simulink model "switch_inductor_system"  (R2025b)
settings: Solver=ode23t  StartTime=0.0  StopTime=10e-6  MaxStep=1e-8  RelTol=1e-4
libraries: fl_lib x93, nesl_utility x82, eeGeneralControl x28, batteryecm_lib x17, eePwmGenerator x11, slpidlib x9, simulink x2, slctrl_fre x1
(part 3 of 3)

== system switch_inductor_system/Feedback_BC6 ==
  u : Inport
  Constant7 : Constant  Value=0.5
  PID Controller1 : slpidlib/PID Controller  Controller=PI  Form=Parallel  TimeDomain=Discrete-time  UseExternalTs=off  SampleTime=1e-5  IntegratorMethod=Forward Euler  FilterMethod=Forward Euler  ControllerParametersSource=internal  P=1  I=3  UseKiTs=off  D=0  UseExternalDerivativeSource=off  N=100  UseFilter=on  TunerSelectOption=Transfer Function Based (PID Tuner App)  InitialConditionSource=internal  InitialConditionForIntegrator=0  InitialConditionForFilter=0  DifferentiatorICPrevScaledInput=0  ExternalReset=none  TrackingMode=off  Kt=1  LimitOutput=on  SatLimitsSource=internal  UpperSaturationLimit=0.5  LowerSaturationLimit=-0.5  LinearizeAsGain=on  AntiWindupMode=clamping  Kb=1  LimitIntegrator=off  UpperIntegratorSaturationLimit=inf  LowerIntegratorSaturationLimit=-inf  POutMin=[]  POutMax=[]  IOutMin=[]  IOutMax=[]  DOutMin=[]  DOutMax=[]  NOutMin=[]  NOutMax=[]  SumOutMin=[]  SumOutMax=[]  SaturationOutMin=[]  SaturationOutMax=[]  PParamMin=[]  PParamMax=[]  IParamMin=[]  IParamMax=[]  DParamMin=[]  DParamMax=[]  NParamMin=[]  NParamMax=[]  KbParamMin=[]  KbParamMax=[]  KtParamMin=[]  KtParamMax=[]  KbOutMin=[]  KbOutMax=[]  KtOutMin=[]  KtOutMax=[]  IntegratorOutMin=[]  IntegratorOutMax=[]  FilterOutMin=[]  FilterOutMax=[]  SumI1OutMin=[]  SumI1OutMax=[]  SumI2OutMin=[]  SumI2OutMax=[]  SumI3OutMin=[]  SumI3OutMax=[]  SumI4OutMin=[]  SumI4OutMax=[]  SumDOutMin=[]  SumDOutMax=[]  DifferentiatorOutMin=[]  DifferentiatorOutMax=[]  FilterDiffOutCoefMin=[]  FilterDiffOutCoefMax=[]  ReciprocalOutMin=[]  ReciprocalOutMax=[]  SumDenOutMin=[]  SumDenOutMax=[]  SumNumOutMin=[]  SumNumOutMax=[]  DivideOutMin=[]  DivideOutMax=[]  UdiffTsProdOutMin=[]  UdiffTsProdOutMax=[]  NTsProdOutMin=[]  NTsProdOutMax=[]  UintegralTsProdOutMin=[]  UintegralTsProdOutMax=[]  UngainTsProdOutMin=[]  UngainTsProdOutMax=[]  ClampingZeroOutDataTypeStr=Inherit: Inherit via back propagation  ClampingZeroOutMin=[]  ClampingZeroOutMax=[]  FilterDenConstantOutDataTypeStr=Inherit: Inherit via back propagation  FilterDenConstantOutMin=[]  FilterDenConstantOutMax=[]  PCopyOutDataTypeStr=Inherit: Inherit via back propagation  PCopyOutMin=[]  PCopyOutMax=[]  NCopyOutDataTypeStr=Inherit: Inherit via back propagation  NCopyOutMin=[]  NCopyOutMax=[]  IntegratorContinuousStateAttributes=''  IntegratorStateMustResolveToSignalObject=off  IntegratorRTWStateStorageClass=Auto  FilterContinuousStateAttributes=''  FilterStateMustResolveToSignalObject=off  FilterRTWStateStorageClass=Auto  ParallelPVariant=InternalParameters  IdealPVariant=Disabled  IVariant=InternalParameters  DVariant=Disabled  IntegratorVariant=Discrete  SatVariant=Enabled  AWVariant=DiscClampingParallel  PCopyVariant=Disabled  TRVariant=Disabled  FdbkBlocksVariant=Forward  IdealPFdbkVariant=Disabled  SatFdbkVariant=Disabled  DerivativeFilterVariant=Disabled  NVariant=Disabled  NCopyVariant=Disabled_SignalSpec  FilterICVariant=Disabled  IntegratorICVariant=InternalICs  ExternalResetVariant=Disabled  TRSumVariant=Passthrough  SumFdbkVariant=Disabled  SumVariant=Sum_PI  TsampFilterVariant=InternalTs  TsampNgainVariant=Passthrough  TsampIntegralVariant=Disabled_SignalSpec  ExternalSaturationOutDataTypeStr=Inherit: Same as second input  DerivativeSourceVariant=Disabled  PreIntVariant=InternalPreInt
  PWM Generator : eePwmGenerator/PWM Generator  CarrCount=Up  Tper=1e-5  Tdelay=0  Ts=1e-8
  Saturation1 : Saturate  UpperLimit=0.8  LowerLimit=0.2
  Scope10 : Scope
      settings: DataLoggingVariableName=ScopeData10
  Scope9 : Scope
      settings: ActiveDisplayYMinimum=0.37658910329171397  ActiveDisplayYMaximum=0.57295686719636774  DataLoggingVariableName=ScopeData9
  Sum7 : Sum  Inputs=|++
  Unit Delay : UnitDelay  InitialCondition=0.5  SampleTime=1e-5  HasFrameUpgradeWarning=on
  PWM : Outport
  wires:
  PID Controller1/1 -> Scope10/1, Sum7/1
  u/1 -> PID Controller1/1
  Constant7/1 -> Sum7/2
  Unit Delay/1 -> Scope9/1, PWM Generator/1
  Saturation1/1 -> Unit Delay/1
  PWM Generator/1 -> PWM/1
  Sum7/1 -> Saturation1/1

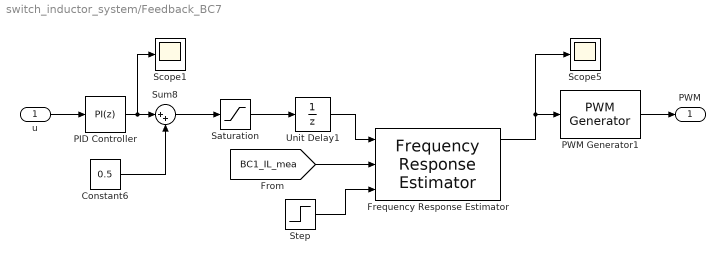
== system switch_inductor_system/Feedback_BC7 ==
  u : Inport
  Constant6 : Constant  Value=0.5
  Frequency Response Estimator : slctrl_fre/Frequency Response Estimator  DiscreteTs=1e-5  OutputMode=control action + perturbation  BlockDataType=double  SineSource=Block parameters  Frequencies=2*pi*logspace(0, 4, 35)  FreqUnits=rad/s  Amplitudes=0.004  NumOfFreq=3  ExperimentMode=Sinestream  NumOfSetPeriod=4  NumOfEstPeriod=6  NumOfSlowestPeriod=3  NumOfPRBSPeriod=1  UseAutogenNumOfPRBSPeriod=off  PRBSSignalOrder=12  UseAutogenPRBSSignalOrder=off  EstimationMode=Online  UseBodePlot=on  BaselinePlant=[]  PlotRefreshFactor=10000  UseExternalTs=off  BodePlotChoice=VariantBode  ExperimentChoice=VariantSS  OutputChoice=VariantCandD  CompiledTsChoice=InternalTs
      settings: LibrarySourceBlock=slctrlblks/Frequency Response Estimation/Frequency Response Estimator
  PID Controller : slpidlib/PID Controller  Controller=PI  Form=Parallel  TimeDomain=Discrete-time  UseExternalTs=off  SampleTime=1e-5  IntegratorMethod=Forward Euler  FilterMethod=Forward Euler  ControllerParametersSource=internal  P=1  I=3  UseKiTs=off  D=0  UseExternalDerivativeSource=off  N=100  UseFilter=on  TunerSelectOption=Transfer Function Based (PID Tuner App)  InitialConditionSource=internal  InitialConditionForIntegrator=0  InitialConditionForFilter=0  DifferentiatorICPrevScaledInput=0  ExternalReset=none  TrackingMode=off  Kt=1  LimitOutput=on  SatLimitsSource=internal  UpperSaturationLimit=0.5  LowerSaturationLimit=-0.5  LinearizeAsGain=on  AntiWindupMode=clamping  Kb=1  LimitIntegrator=off  UpperIntegratorSaturationLimit=inf  LowerIntegratorSaturationLimit=-inf  POutMin=[]  POutMax=[]  IOutMin=[]  IOutMax=[]  DOutMin=[]  DOutMax=[]  NOutMin=[]  NOutMax=[]  SumOutMin=[]  SumOutMax=[]  SaturationOutMin=[]  SaturationOutMax=[]  PParamMin=[]  PParamMax=[]  IParamMin=[]  IParamMax=[]  DParamMin=[]  DParamMax=[]  NParamMin=[]  NParamMax=[]  KbParamMin=[]  KbParamMax=[]  KtParamMin=[]  KtParamMax=[]  KbOutMin=[]  KbOutMax=[]  KtOutMin=[]  KtOutMax=[]  IntegratorOutMin=[]  IntegratorOutMax=[]  FilterOutMin=[]  FilterOutMax=[]  SumI1OutMin=[]  SumI1OutMax=[]  SumI2OutMin=[]  SumI2OutMax=[]  SumI3OutMin=[]  SumI3OutMax=[]  SumI4OutMin=[]  SumI4OutMax=[]  SumDOutMin=[]  SumDOutMax=[]  DifferentiatorOutMin=[]  DifferentiatorOutMax=[]  FilterDiffOutCoefMin=[]  FilterDiffOutCoefMax=[]  ReciprocalOutMin=[]  ReciprocalOutMax=[]  SumDenOutMin=[]  SumDenOutMax=[]  SumNumOutMin=[]  SumNumOutMax=[]  DivideOutMin=[]  DivideOutMax=[]  UdiffTsProdOutMin=[]  UdiffTsProdOutMax=[]  NTsProdOutMin=[]  NTsProdOutMax=[]  UintegralTsProdOutMin=[]  UintegralTsProdOutMax=[]  UngainTsProdOutMin=[]  UngainTsProdOutMax=[]  ClampingZeroOutDataTypeStr=Inherit: Inherit via back propagation  ClampingZeroOutMin=[]  ClampingZeroOutMax=[]  FilterDenConstantOutDataTypeStr=Inherit: Inherit via back propagation  FilterDenConstantOutMin=[]  FilterDenConstantOutMax=[]  PCopyOutDataTypeStr=Inherit: Inherit via back propagation  PCopyOutMin=[]  PCopyOutMax=[]  NCopyOutDataTypeStr=Inherit: Inherit via back propagation  NCopyOutMin=[]  NCopyOutMax=[]  IntegratorContinuousStateAttributes=''  IntegratorStateMustResolveToSignalObject=off  IntegratorRTWStateStorageClass=Auto  FilterContinuousStateAttributes=''  FilterStateMustResolveToSignalObject=off  FilterRTWStateStorageClass=Auto  ParallelPVariant=InternalParameters  IdealPVariant=Disabled  IVariant=InternalParameters  DVariant=Disabled  IntegratorVariant=Discrete  SatVariant=Enabled  AWVariant=DiscClampingParallel  PCopyVariant=Disabled  TRVariant=Disabled  FdbkBlocksVariant=Forward  IdealPFdbkVariant=Disabled  SatFdbkVariant=Disabled  DerivativeFilterVariant=Disabled  NVariant=Disabled  NCopyVariant=Disabled_SignalSpec  FilterICVariant=Disabled  IntegratorICVariant=InternalICs  ExternalResetVariant=Disabled  TRSumVariant=Passthrough  SumFdbkVariant=Disabled  SumVariant=Sum_PI  TsampFilterVariant=InternalTs  TsampNgainVariant=Passthrough  TsampIntegralVariant=Disabled_SignalSpec  ExternalSaturationOutDataTypeStr=Inherit: Same as second input  DerivativeSourceVariant=Disabled  PreIntVariant=InternalPreInt
  PWM Generator1 : eePwmGenerator/PWM Generator  CarrCount=Up  Tper=1e-5  Tdelay=0  Ts=1e-8
  Saturation : Saturate  UpperLimit=0.8  LowerLimit=0.2
  Scope1 : Scope
      settings: ActiveDisplayYMinimum=-0.042552531642600082  ActiveDisplayYMaximum=0.10471177602951695
  Scope5 : Scope
      settings: ActiveDisplayYMinimum=0.39070761591509251  ActiveDisplayYMaximum=0.50905716116304278  DataLoggingVariableName=ScopeData3
  Step : Step  Time=0.5  SampleTime=0
  Sum8 : Sum  Inputs=|++
  Unit Delay1 : UnitDelay  InitialCondition=0.5  SampleTime=1e-5  HasFrameUpgradeWarning=on
  PWM : Outport
  wires:
  Sum8/1 -> Saturation/1
  PID Controller/1 -> Scope1/1, Sum8/1
  Constant6/1 -> Sum8/2
  Saturation/1 -> Unit Delay1/1
  u/1 -> PID Controller/1
  PWM Generator1/1 -> PWM/1
  Unit Delay1/1 -> Frequency Response Estimator/1
  Frequency Response Estimator/1 -> Scope5/1, PWM Generator1/1
  [BC1_IL_mea] -> Frequency Response Estimator/2
  Step/1 -> Frequency Response Estimator/3

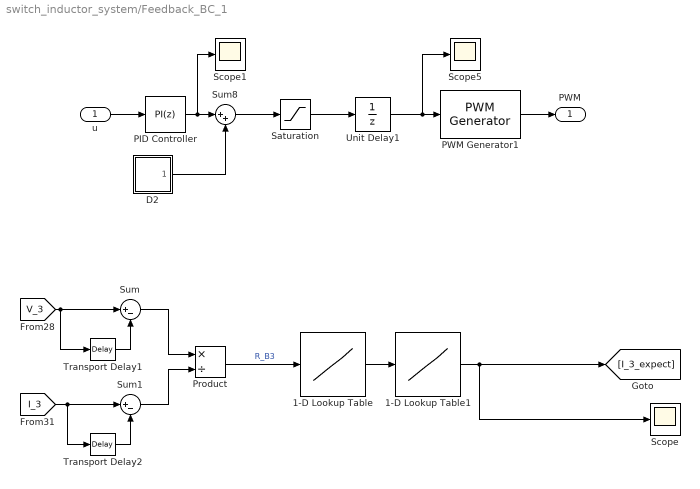
== system switch_inductor_system/Feedback_BC_1 ==
  u : Inport
  1-D Lookup Table : Lookup_n-D  NumberOfTableDimensions=1  BreakpointsForDimension1=[0.005 0.0055 0.006 0.0065 0.007 0.0075 0.008 0.008500000000000001 0.008999999999999999 0.0095 0.01]  Table=[100 90 80 70 60 50 40 30 20 10 5]  InternalRulePriority=Speed  RndMeth=Simplest
  1-D Lookup Table1 : Lookup_n-D  NumberOfTableDimensions=1  BreakpointsForDimension1=[5 10 20 30 40 50 60 70 80 90 100]  Table=[0.6 0.7 0.7125 0.725 0.75 0.8 0.9 1 1.1 1.2 1.3]  InternalRulePriority=Speed  RndMeth=Simplest
  D2 : Subsystem
  PID Controller : slpidlib/PID Controller  Controller=PI  Form=Parallel  TimeDomain=Discrete-time  UseExternalTs=off  SampleTime=1e-5  IntegratorMethod=Forward Euler  FilterMethod=Forward Euler  ControllerParametersSource=internal  P=1  I=3  UseKiTs=off  D=0  UseExternalDerivativeSource=off  N=100  UseFilter=on  TunerSelectOption=Transfer Function Based (PID Tuner App)  InitialConditionSource=internal  InitialConditionForIntegrator=0  InitialConditionForFilter=0  DifferentiatorICPrevScaledInput=0  ExternalReset=none  TrackingMode=off  Kt=1  LimitOutput=on  SatLimitsSource=internal  UpperSaturationLimit=0.5  LowerSaturationLimit=-0.5  LinearizeAsGain=on  AntiWindupMode=clamping  Kb=1  LimitIntegrator=off  UpperIntegratorSaturationLimit=inf  LowerIntegratorSaturationLimit=-inf  POutMin=[]  POutMax=[]  IOutMin=[]  IOutMax=[]  DOutMin=[]  DOutMax=[]  NOutMin=[]  NOutMax=[]  SumOutMin=[]  SumOutMax=[]  SaturationOutMin=[]  SaturationOutMax=[]  PParamMin=[]  PParamMax=[]  IParamMin=[]  IParamMax=[]  DParamMin=[]  DParamMax=[]  NParamMin=[]  NParamMax=[]  KbParamMin=[]  KbParamMax=[]  KtParamMin=[]  KtParamMax=[]  KbOutMin=[]  KbOutMax=[]  KtOutMin=[]  KtOutMax=[]  IntegratorOutMin=[]  IntegratorOutMax=[]  FilterOutMin=[]  FilterOutMax=[]  SumI1OutMin=[]  SumI1OutMax=[]  SumI2OutMin=[]  SumI2OutMax=[]  SumI3OutMin=[]  SumI3OutMax=[]  SumI4OutMin=[]  SumI4OutMax=[]  SumDOutMin=[]  SumDOutMax=[]  DifferentiatorOutMin=[]  DifferentiatorOutMax=[]  FilterDiffOutCoefMin=[]  FilterDiffOutCoefMax=[]  ReciprocalOutMin=[]  ReciprocalOutMax=[]  SumDenOutMin=[]  SumDenOutMax=[]  SumNumOutMin=[]  SumNumOutMax=[]  DivideOutMin=[]  DivideOutMax=[]  UdiffTsProdOutMin=[]  UdiffTsProdOutMax=[]  NTsProdOutMin=[]  NTsProdOutMax=[]  UintegralTsProdOutMin=[]  UintegralTsProdOutMax=[]  UngainTsProdOutMin=[]  UngainTsProdOutMax=[]  ClampingZeroOutDataTypeStr=Inherit: Inherit via back propagation  ClampingZeroOutMin=[]  ClampingZeroOutMax=[]  FilterDenConstantOutDataTypeStr=Inherit: Inherit via back propagation  FilterDenConstantOutMin=[]  FilterDenConstantOutMax=[]  PCopyOutDataTypeStr=Inherit: Inherit via back propagation  PCopyOutMin=[]  PCopyOutMax=[]  NCopyOutDataTypeStr=Inherit: Inherit via back propagation  NCopyOutMin=[]  NCopyOutMax=[]  IntegratorContinuousStateAttributes=''  IntegratorStateMustResolveToSignalObject=off  IntegratorRTWStateStorageClass=Auto  FilterContinuousStateAttributes=''  FilterStateMustResolveToSignalObject=off  FilterRTWStateStorageClass=Auto  ParallelPVariant=InternalParameters  IdealPVariant=Disabled  IVariant=InternalParameters  DVariant=Disabled  IntegratorVariant=Discrete  SatVariant=Enabled  AWVariant=DiscClampingParallel  PCopyVariant=Disabled  TRVariant=Disabled  FdbkBlocksVariant=Forward  IdealPFdbkVariant=Disabled  SatFdbkVariant=Disabled  DerivativeFilterVariant=Disabled  NVariant=Disabled  NCopyVariant=Disabled_SignalSpec  FilterICVariant=Disabled  IntegratorICVariant=InternalICs  ExternalResetVariant=Disabled  TRSumVariant=Passthrough  SumFdbkVariant=Disabled  SumVariant=Sum_PI  TsampFilterVariant=InternalTs  TsampNgainVariant=Passthrough  TsampIntegralVariant=Disabled_SignalSpec  ExternalSaturationOutDataTypeStr=Inherit: Same as second input  DerivativeSourceVariant=Disabled  PreIntVariant=InternalPreInt
  PWM Generator1 : eePwmGenerator/PWM Generator  CarrCount=Up  Tper=1e-5  Tdelay=0  Ts=1e-8
  Product : Product  Inputs=*/
  Saturation : Saturate  UpperLimit=0.8  LowerLimit=0.2
  Scope : Scope
      settings: ActiveDisplayYMinimum=-2.9852928329645325E+11  ActiveDisplayYMaximum=4.8687718951302284E+10  DataLoggingVariableName=ScopeData13
  Scope1 : Scope
      settings: ActiveDisplayYMinimum=-0.1509051118952274  ActiveDisplayYMaximum=0.35121566965953643
  Scope5 : Scope
      settings: ActiveDisplayYMinimum=0.39070761591509251  ActiveDisplayYMaximum=0.50905716116304278  DataLoggingVariableName=ScopeData3
  Sum : Sum  Inputs=|+-
  Sum1 : Sum  Inputs=|+-
  Sum8 : Sum  Inputs=|++
  Transport Delay1 : TransportDelay  DelayTime=0.01
  Transport Delay2 : TransportDelay  DelayTime=0.01
  Unit Delay1 : UnitDelay  InitialCondition=0.5  SampleTime=1e-5  HasFrameUpgradeWarning=on
  PWM : Outport
  wires:
  Unit Delay1/1 -> Scope5/1, PWM Generator1/1
  Sum8/1 -> Saturation/1
  PID Controller/1 -> Scope1/1, Sum8/1
  D2/1(Out1) -> Sum8/2
  Saturation/1 -> Unit Delay1/1
  u/1 -> PID Controller/1
  PWM Generator1/1 -> PWM/1
  [V_3] -> Sum/1, Transport Delay1/1
  Transport Delay1/1 -> Sum/2
  [I_3] -> Transport Delay2/1, Sum1/1
  Transport Delay2/1 -> Sum1/2
  Sum/1 -> Product/1
  Sum1/1 -> Product/2
  Product/1 -> 1-D Lookup Table/1  "R_B3"
  1-D Lookup Table/1 -> 1-D Lookup Table1/1
  1-D Lookup Table1/1 -> Scope/1, [I_3_expect]

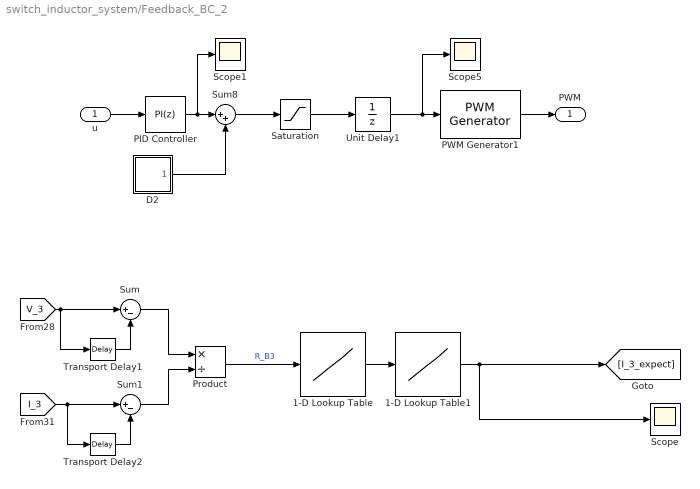
== system switch_inductor_system/Feedback_BC_2 ==
  u : Inport
  1-D Lookup Table : Lookup_n-D  NumberOfTableDimensions=1  BreakpointsForDimension1=[0.005 0.0055 0.006 0.0065 0.007 0.0075 0.008 0.008500000000000001 0.008999999999999999 0.0095 0.01]  Table=[100 90 80 70 60 50 40 30 20 10 5]  InternalRulePriority=Speed  RndMeth=Simplest
  1-D Lookup Table1 : Lookup_n-D  NumberOfTableDimensions=1  BreakpointsForDimension1=[5 10 20 30 40 50 60 70 80 90 100]  Table=[0.6 0.7 0.7125 0.725 0.75 0.8 0.9 1 1.1 1.2 1.3]  InternalRulePriority=Speed  RndMeth=Simplest
  D2 : Subsystem
  PID Controller : slpidlib/PID Controller  Controller=PI  Form=Parallel  TimeDomain=Discrete-time  UseExternalTs=off  SampleTime=1e-5  IntegratorMethod=Forward Euler  FilterMethod=Forward Euler  ControllerParametersSource=internal  P=1  I=3  UseKiTs=off  D=0  UseExternalDerivativeSource=off  N=100  UseFilter=on  TunerSelectOption=Transfer Function Based (PID Tuner App)  InitialConditionSource=internal  InitialConditionForIntegrator=0  InitialConditionForFilter=0  DifferentiatorICPrevScaledInput=0  ExternalReset=none  TrackingMode=off  Kt=1  LimitOutput=on  SatLimitsSource=internal  UpperSaturationLimit=0.5  LowerSaturationLimit=-0.5  LinearizeAsGain=on  AntiWindupMode=clamping  Kb=1  LimitIntegrator=off  UpperIntegratorSaturationLimit=inf  LowerIntegratorSaturationLimit=-inf  POutMin=[]  POutMax=[]  IOutMin=[]  IOutMax=[]  DOutMin=[]  DOutMax=[]  NOutMin=[]  NOutMax=[]  SumOutMin=[]  SumOutMax=[]  SaturationOutMin=[]  SaturationOutMax=[]  PParamMin=[]  PParamMax=[]  IParamMin=[]  IParamMax=[]  DParamMin=[]  DParamMax=[]  NParamMin=[]  NParamMax=[]  KbParamMin=[]  KbParamMax=[]  KtParamMin=[]  KtParamMax=[]  KbOutMin=[]  KbOutMax=[]  KtOutMin=[]  KtOutMax=[]  IntegratorOutMin=[]  IntegratorOutMax=[]  FilterOutMin=[]  FilterOutMax=[]  SumI1OutMin=[]  SumI1OutMax=[]  SumI2OutMin=[]  SumI2OutMax=[]  SumI3OutMin=[]  SumI3OutMax=[]  SumI4OutMin=[]  SumI4OutMax=[]  SumDOutMin=[]  SumDOutMax=[]  DifferentiatorOutMin=[]  DifferentiatorOutMax=[]  FilterDiffOutCoefMin=[]  FilterDiffOutCoefMax=[]  ReciprocalOutMin=[]  ReciprocalOutMax=[]  SumDenOutMin=[]  SumDenOutMax=[]  SumNumOutMin=[]  SumNumOutMax=[]  DivideOutMin=[]  DivideOutMax=[]  UdiffTsProdOutMin=[]  UdiffTsProdOutMax=[]  NTsProdOutMin=[]  NTsProdOutMax=[]  UintegralTsProdOutMin=[]  UintegralTsProdOutMax=[]  UngainTsProdOutMin=[]  UngainTsProdOutMax=[]  ClampingZeroOutDataTypeStr=Inherit: Inherit via back propagation  ClampingZeroOutMin=[]  ClampingZeroOutMax=[]  FilterDenConstantOutDataTypeStr=Inherit: Inherit via back propagation  FilterDenConstantOutMin=[]  FilterDenConstantOutMax=[]  PCopyOutDataTypeStr=Inherit: Inherit via back propagation  PCopyOutMin=[]  PCopyOutMax=[]  NCopyOutDataTypeStr=Inherit: Inherit via back propagation  NCopyOutMin=[]  NCopyOutMax=[]  IntegratorContinuousStateAttributes=''  IntegratorStateMustResolveToSignalObject=off  IntegratorRTWStateStorageClass=Auto  FilterContinuousStateAttributes=''  FilterStateMustResolveToSignalObject=off  FilterRTWStateStorageClass=Auto  ParallelPVariant=InternalParameters  IdealPVariant=Disabled  IVariant=InternalParameters  DVariant=Disabled  IntegratorVariant=Discrete  SatVariant=Enabled  AWVariant=DiscClampingParallel  PCopyVariant=Disabled  TRVariant=Disabled  FdbkBlocksVariant=Forward  IdealPFdbkVariant=Disabled  SatFdbkVariant=Disabled  DerivativeFilterVariant=Disabled  NVariant=Disabled  NCopyVariant=Disabled_SignalSpec  FilterICVariant=Disabled  IntegratorICVariant=InternalICs  ExternalResetVariant=Disabled  TRSumVariant=Passthrough  SumFdbkVariant=Disabled  SumVariant=Sum_PI  TsampFilterVariant=InternalTs  TsampNgainVariant=Passthrough  TsampIntegralVariant=Disabled_SignalSpec  ExternalSaturationOutDataTypeStr=Inherit: Same as second input  DerivativeSourceVariant=Disabled  PreIntVariant=InternalPreInt
  PWM Generator1 : eePwmGenerator/PWM Generator  CarrCount=Up  Tper=1e-5  Tdelay=0  Ts=1e-8
  Product : Product  Inputs=*/
  Saturation : Saturate  UpperLimit=0.8  LowerLimit=0.2
  Scope : Scope
      settings: ActiveDisplayYMinimum=-2.9852928329645325E+11  ActiveDisplayYMaximum=4.8687718951302284E+10  DataLoggingVariableName=ScopeData13
  Scope1 : Scope
      settings: ActiveDisplayYMinimum=-0.1509051118952274  ActiveDisplayYMaximum=0.35121566965953643
  Scope5 : Scope
      settings: ActiveDisplayYMinimum=0.39070761591509251  ActiveDisplayYMaximum=0.50905716116304278  DataLoggingVariableName=ScopeData3
  Sum : Sum  Inputs=|+-
  Sum1 : Sum  Inputs=|+-
  Sum8 : Sum  Inputs=|++
  Transport Delay1 : TransportDelay  DelayTime=0.01
  Transport Delay2 : TransportDelay  DelayTime=0.01
  Unit Delay1 : UnitDelay  InitialCondition=0.5  SampleTime=1e-5  HasFrameUpgradeWarning=on
  PWM : Outport
  wires:
  Unit Delay1/1 -> Scope5/1, PWM Generator1/1
  Sum8/1 -> Saturation/1
  PID Controller/1 -> Scope1/1, Sum8/1
  D2/1(Out1) -> Sum8/2
  Saturation/1 -> Unit Delay1/1
  u/1 -> PID Controller/1
  PWM Generator1/1 -> PWM/1
  [V_3] -> Sum/1, Transport Delay1/1
  Transport Delay1/1 -> Sum/2
  [I_3] -> Transport Delay2/1, Sum1/1
  Transport Delay2/1 -> Sum1/2
  Sum/1 -> Product/1
  Sum1/1 -> Product/2
  Product/1 -> 1-D Lookup Table/1  "R_B3"
  1-D Lookup Table/1 -> 1-D Lookup Table1/1
  1-D Lookup Table1/1 -> Scope/1, [I_3_expect]

== system switch_inductor_system/Lambda_BC1 ==
  In1 : Inport
  Abs : Abs  SaturateOnIntegerOverflow=off
  Data Type Conversion : DataTypeConversion  SaturateOnIntegerOverflow=off  RndMeth=Floor
  Relational Operator2 : RelationalOperator  Operator=>  OutDataTypeStr=boolean  RndMeth=Simplest  InputSameDT=off
  V_th2 : Constant  Value=0.01
  Lambda_BC1 : Outport
  wires:
  Relational Operator2/1 -> Data Type Conversion/1
  Abs/1 -> Relational Operator2/1
  V_th2/1 -> Relational Operator2/2
  Data Type Conversion/1 -> Lambda_BC1/1  "Lambda_BC1"
  In1/1 -> Abs/1

== system switch_inductor_system/Lambda_BC2 ==
  In1 : Inport
  Abs1 : Abs  SaturateOnIntegerOverflow=off
  Data Type Conversion3 : DataTypeConversion  SaturateOnIntegerOverflow=off  RndMeth=Floor
  Relational Operator1 : RelationalOperator  Operator=>  OutDataTypeStr=boolean  RndMeth=Simplest  InputSameDT=off
  V_th1 : Constant  Value=0.01
  Lambda_BC2 : Outport
  wires:
  Abs1/1 -> Relational Operator1/1
  V_th1/1 -> Relational Operator1/2
  Relational Operator1/1 -> Data Type Conversion3/1
  Data Type Conversion3/1 -> Lambda_BC2/1  "Lambda_BC2"
  In1/1 -> Abs1/1

== system switch_inductor_system/Lambda_BC3 ==
  In1 : Inport
  Abs : Abs  SaturateOnIntegerOverflow=off
  Data Type Conversion : DataTypeConversion  SaturateOnIntegerOverflow=off  RndMeth=Floor
  Relational Operator2 : RelationalOperator  Operator=>  OutDataTypeStr=boolean  RndMeth=Simplest  InputSameDT=off
  V_th2 : Constant  Value=0.01
  Lambda_BC1 : Outport
  wires:
  Relational Operator2/1 -> Data Type Conversion/1
  Abs/1 -> Relational Operator2/1
  V_th2/1 -> Relational Operator2/2
  Data Type Conversion/1 -> Lambda_BC1/1  "Lambda_BC1"
  In1/1 -> Abs/1

== system switch_inductor_system/Lambda_BC4 ==
  In1 : Inport
  Abs1 : Abs  SaturateOnIntegerOverflow=off
  Data Type Conversion3 : DataTypeConversion  SaturateOnIntegerOverflow=off  RndMeth=Floor
  Relational Operator1 : RelationalOperator  Operator=>  OutDataTypeStr=boolean  RndMeth=Simplest  InputSameDT=off
  V_th1 : Constant  Value=0.01
  Lambda_BC2 : Outport
  wires:
  Abs1/1 -> Relational Operator1/1
  V_th1/1 -> Relational Operator1/2
  Relational Operator1/1 -> Data Type Conversion3/1
  Data Type Conversion3/1 -> Lambda_BC2/1  "Lambda_BC2"
  In1/1 -> Abs1/1

== system switch_inductor_system/Lambda_BC5 ==
  In1 : Inport
  Abs : Abs  SaturateOnIntegerOverflow=off
  Data Type Conversion : DataTypeConversion  SaturateOnIntegerOverflow=off  RndMeth=Floor
  Relational Operator2 : RelationalOperator  Operator=>  OutDataTypeStr=boolean  RndMeth=Simplest  InputSameDT=off
  V_th2 : Constant  Value=0.01
  Lambda_BC1 : Outport
  wires:
  Relational Operator2/1 -> Data Type Conversion/1
  Abs/1 -> Relational Operator2/1
  V_th2/1 -> Relational Operator2/2
  Data Type Conversion/1 -> Lambda_BC1/1  "Lambda_BC1"
  In1/1 -> Abs/1

== system switch_inductor_system/Lambda_BC6 ==
  In1 : Inport
  Abs : Abs  SaturateOnIntegerOverflow=off
  Data Type Conversion : DataTypeConversion  SaturateOnIntegerOverflow=off  RndMeth=Floor
  Relational Operator2 : RelationalOperator  Operator=>  OutDataTypeStr=boolean  RndMeth=Simplest  InputSameDT=off
  V_th2 : Constant  Value=0.01
  Lambda_BC1 : Outport
  wires:
  Relational Operator2/1 -> Data Type Conversion/1
  Abs/1 -> Relational Operator2/1
  V_th2/1 -> Relational Operator2/2
  Data Type Conversion/1 -> Lambda_BC1/1  "Lambda_BC1"
  In1/1 -> Abs/1

== system switch_inductor_system/Lambda_BC7 ==
  In1 : Inport
  Abs1 : Abs  SaturateOnIntegerOverflow=off
  Data Type Conversion3 : DataTypeConversion  SaturateOnIntegerOverflow=off  RndMeth=Floor
  Relational Operator1 : RelationalOperator  Operator=>  OutDataTypeStr=boolean  RndMeth=Simplest  InputSameDT=off
  V_th1 : Constant  Value=0.01
  Lambda_BC2 : Outport
  wires:
  Abs1/1 -> Relational Operator1/1
  V_th1/1 -> Relational Operator1/2
  Relational Operator1/1 -> Data Type Conversion3/1
  Data Type Conversion3/1 -> Lambda_BC2/1  "Lambda_BC2"
  In1/1 -> Abs1/1

== system switch_inductor_system/Lambda_BC8 ==
  In1 : Inport
  Abs : Abs  SaturateOnIntegerOverflow=off
  Data Type Conversion : DataTypeConversion  SaturateOnIntegerOverflow=off  RndMeth=Floor
  Relational Operator2 : RelationalOperator  Operator=>  OutDataTypeStr=boolean  RndMeth=Simplest  InputSameDT=off
  V_th2 : Constant  Value=0.01
  Lambda_BC1 : Outport
  wires:
  Relational Operator2/1 -> Data Type Conversion/1
  Abs/1 -> Relational Operator2/1
  V_th2/1 -> Relational Operator2/2
  Data Type Conversion/1 -> Lambda_BC1/1  "Lambda_BC1"
  In1/1 -> Abs/1

== system switch_inductor_system/Lambda_BC9 ==
  In1 : Inport
  Abs1 : Abs  SaturateOnIntegerOverflow=off
  Data Type Conversion3 : DataTypeConversion  SaturateOnIntegerOverflow=off  RndMeth=Floor
  Relational Operator1 : RelationalOperator  Operator=>  OutDataTypeStr=boolean  RndMeth=Simplest  InputSameDT=off
  V_th1 : Constant  Value=0.01
  Lambda_BC2 : Outport
  wires:
  Abs1/1 -> Relational Operator1/1
  V_th1/1 -> Relational Operator1/2
  Relational Operator1/1 -> Data Type Conversion3/1
  Data Type Conversion3/1 -> Lambda_BC2/1  "Lambda_BC2"
  In1/1 -> Abs1/1

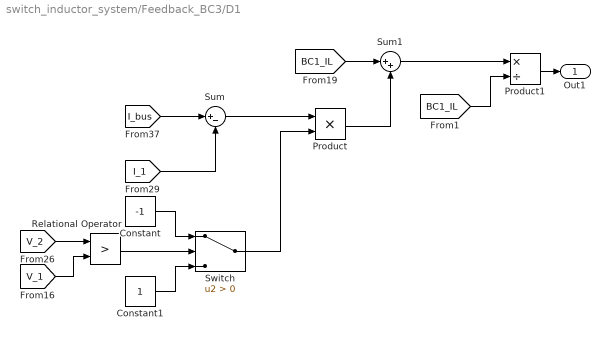
== system switch_inductor_system/Feedback_BC3/D1 ==
  Constant : Constant  Value=-1
  Constant1 : Constant
  Product : Product
  Product1 : Product  Inputs=*/
  Relational Operator : RelationalOperator  Operator=>  OutDataTypeStr=boolean  RndMeth=Simplest  InputSameDT=off
  Sum : Sum  Inputs=|+-
  Sum1 : Sum  Inputs=|++
  Switch : Switch  Criteria=u2 > Threshold  SaturateOnIntegerOverflow=off  InputSameDT=off
  Out1 : Outport
  wires:
  Product1/1 -> Out1/1
  [BC1_IL] -> Sum1/1
  Sum/1 -> Product/1
  Constant1/1 -> Switch/3
  [BC1_IL] -> Product1/2
  [V_1] -> Relational Operator/2
  Relational Operator/1 -> Switch/2
  Sum1/1 -> Product1/1
  Constant/1 -> Switch/1
  Switch/1 -> Product/2
  [I_1] -> Sum/2
  [I_bus] -> Sum/1
  [V_2] -> Relational Operator/1
  Product/1 -> Sum1/2

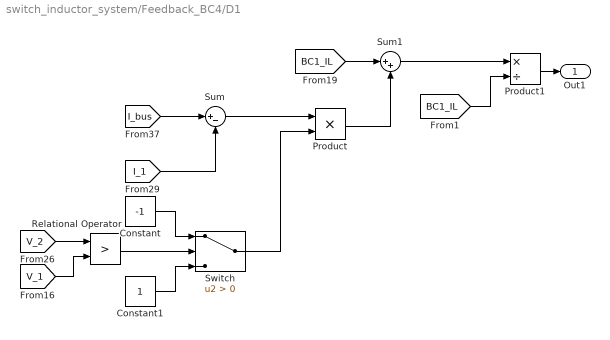
== system switch_inductor_system/Feedback_BC4/D1 ==
  Constant : Constant  Value=-1
  Constant1 : Constant
  Product : Product
  Product1 : Product  Inputs=*/
  Relational Operator : RelationalOperator  Operator=>  OutDataTypeStr=boolean  RndMeth=Simplest  InputSameDT=off
  Sum : Sum  Inputs=|+-
  Sum1 : Sum  Inputs=|++
  Switch : Switch  Criteria=u2 > Threshold  SaturateOnIntegerOverflow=off  InputSameDT=off
  Out1 : Outport
  wires:
  Product1/1 -> Out1/1
  [BC1_IL] -> Sum1/1
  Sum/1 -> Product/1
  Constant1/1 -> Switch/3
  [BC1_IL] -> Product1/2
  [V_1] -> Relational Operator/2
  Relational Operator/1 -> Switch/2
  Sum1/1 -> Product1/1
  Constant/1 -> Switch/1
  Switch/1 -> Product/2
  [I_1] -> Sum/2
  [I_bus] -> Sum/1
  [V_2] -> Relational Operator/1
  Product/1 -> Sum1/2

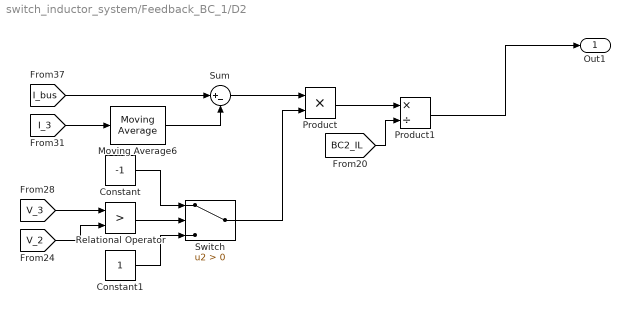
== system switch_inductor_system/Feedback_BC_1/D2 ==
  Constant : Constant  Value=-1
  Constant1 : Constant
  Moving Average6 : eeGeneralControl/Moving Average  VariantControl=Variant1  LabelModeActiveChoice=Discrete  f=1e5  x0=0  BufferSize=8192  Ts=1e-7
      settings: LibrarySourceBlock=ee_sl_lib/General Control/Moving Average
  Product : Product
  Product1 : Product  Inputs=*/
  Relational Operator : RelationalOperator  Operator=>  OutDataTypeStr=boolean  RndMeth=Simplest  InputSameDT=off
  Sum : Sum  Inputs=|+-
  Switch : Switch  Criteria=u2 > Threshold  SaturateOnIntegerOverflow=off  InputSameDT=off
  Out1 : Outport
  wires:
  Switch/1 -> Product/2
  [I_bus] -> Sum/1
  Sum/1 -> Product/1
  Product/1 -> Product1/1
  Constant/1 -> Switch/1
  [I_3] -> Moving Average6/1
  [BC2_IL] -> Product1/2
  Constant1/1 -> Switch/3
  [V_2] -> Relational Operator/2
  [V_3] -> Relational Operator/1
  Relational Operator/1 -> Switch/2
  Product1/1 -> Out1/1
  Moving Average6/1 -> Sum/2

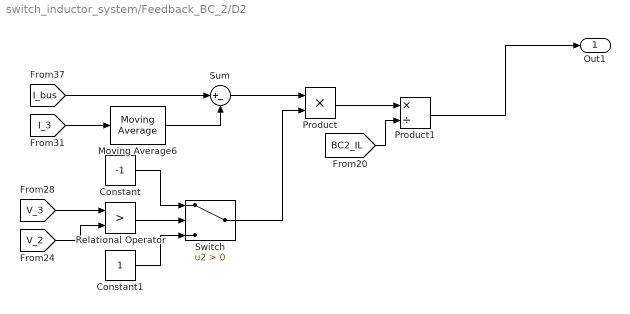
== system switch_inductor_system/Feedback_BC_2/D2 ==
  Constant : Constant  Value=-1
  Constant1 : Constant
  Moving Average6 : eeGeneralControl/Moving Average  VariantControl=Variant1  LabelModeActiveChoice=Discrete  f=1e5  x0=0  BufferSize=8192  Ts=1e-7
      settings: LibrarySourceBlock=ee_sl_lib/General Control/Moving Average
  Product : Product
  Product1 : Product  Inputs=*/
  Relational Operator : RelationalOperator  Operator=>  OutDataTypeStr=boolean  RndMeth=Simplest  InputSameDT=off
  Sum : Sum  Inputs=|+-
  Switch : Switch  Criteria=u2 > Threshold  SaturateOnIntegerOverflow=off  InputSameDT=off
  Out1 : Outport
  wires:
  Switch/1 -> Product/2
  [I_bus] -> Sum/1
  Sum/1 -> Product/1
  Product/1 -> Product1/1
  Constant/1 -> Switch/1
  [I_3] -> Moving Average6/1
  [BC2_IL] -> Product1/2
  Constant1/1 -> Switch/3
  [V_2] -> Relational Operator/2
  [V_3] -> Relational Operator/1
  Relational Operator/1 -> Switch/2
  Product1/1 -> Out1/1
  Moving Average6/1 -> Sum/2
